simulink model "zynq_7000_tutorial_3"  (R2022a)
settings: Solver=FixedStepDiscrete  StartTime=0.0  StopTime=10.0  RelTol=1e-3
PostLoadFcn:
  | zynq7000.setModelProperties(bdroot)
undefined symbols (not defined in the file): AXI_VDMA, B, cam_init, G, init_cam, out1, out2, out3, OV5640, PS_GPIO, PS_IIC, R, read_cam_rgb, ScuGicInterruptController, VideoOutput
libraries: waijung2_utilities_lib x2, deeplib x1
Description:
  | This model is created using Waijung 2
  | (Version: 23.5a)
settings Model: Creator=Aimagin  LastModifiedBy=Chris
settings SolverCC: PositivePriorityOrder=on  AutoInsertRateTranBlk=on
settings OptimizationCC: DefaultParameterBehavior=Inlined  EnhancedBackFolding=on  PassReuseOutputArgsAs=Individual arguments  ZeroExternalMemoryAtStartup=off  ZeroInternalMemoryAtStartup=off  OptimizeBlockOrder=speed  DifferentSizesBufferReuse=on  OptimizationCustomize=off  EfficientTunableParamExpr=on
settings DebuggingCC: ParameterTunabilityLossMsg=error
settings HardwareCC: ProdBitPerPointer=32  ProdBitPerSizeT=32  ProdBitPerPtrDiffT=32  ProdLargestAtomicInteger=Long  ProdLargestAtomicFloat=Double  ProdWordSize=32  ProdHWDeviceType=ARM Compatible->ARM Cortex
settings SFSimCC: MATLABDynamicMemAlloc=off
settings RTWCC: Description=Waijung 2 ZYNQ7000 target  SystemTargetFile=zynq7000.tlc  TemplateMakefile=zynq7000.tmf  RetainRTWFile=on  TargetLang=C++  DLTargetLibrary=arm-compute  DLArmComputeArch=armv7
settings CodeAppCC: ForceParamTrailComments=on  IgnoreCustomStorageClasses=off  OperatorAnnotations=on  SimulinkDataObjDesc=on  SFDataObjDesc=on  InsertBlockDesc=on
settings STFCustomTargetCC: TargetLangStandard=C99 (ISO)  MultiwordLength=256  ModelReferenceCompliant=off  CombineOutputUpdateFcns=on  ERTCustomFileBanners=on  SupportContinuousTime=off  SupportNonInlinedSFcns=off  RemoveResetFunc=on  SupportVariableSizeSignals=on  MATLABClassNameForMDSCustomization=Simulink.SoftwareTarget.ERTCustomization  GRTInterface=off  SystemTargetFile=zynq7000.tlc
settings ERTTargetCC: TargetLangStandard=C99 (ISO)  ModelReferenceCompliant=off  ParMdlRefBuildCompliant=off  CompOptLevelCompliant=off  ConcurrentExecutionCompliant=off  SupportVariableSizeSignals=on  ModelStepFunctionPrototypeControlCompliant=off  CPPClassGenCompliant=off  UseToolchainInfoCompliant=off  InlinedParameterPlacement=NonHierarchical  ERTSrcFileBannerTemplate=zynq7000_code_template.cgt  ERTHdrFileBannerTemplate=zynq7000_code_template.cgt  ERTDataSrcFileTemplate=zynq7000_code_template.cgt  ERTDataHdrFileTemplate=zynq7000_code_template.cgt  ERTCustomFileTemplate=zynq7000_file_process.tlc

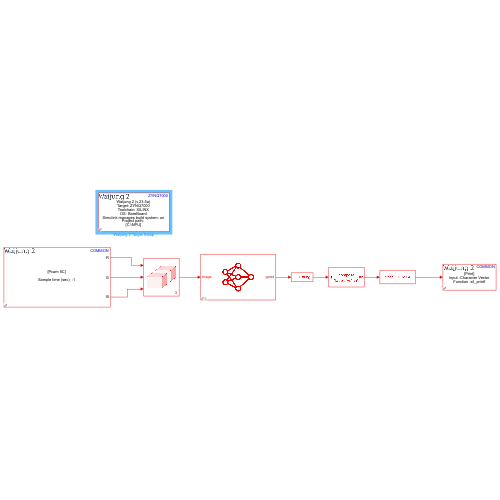
[thumbnail: Simulink's stored preview of the top-level diagram]
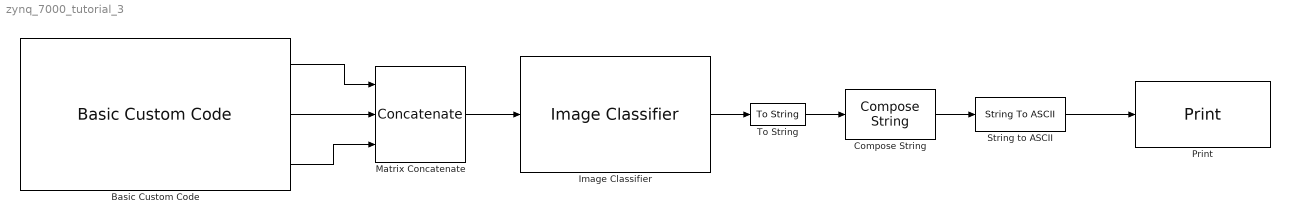
== system zynq_7000_tutorial_3 ==
  Basic Custom Code : waijung2_utilities_lib/Basic Custom Code  blockid=BasicCustomCode  maskdispname=Pcam 5C  inporttable={}  outporttable={ 'R', 'uint8', '1280x720'; 'G', 'uint8', '1280x720'; 'B', 'uint8', '1280x720' }  inputporttype=""  cinputportlabelstr="[\"\"]"  inputportcount=0  inputporttypeid=[-1]  outputporttype=uint8:1280x720,uint8:1280x720,uint8:1280x720  coutputportlabel=R,G,B  coutputportlabelstr="[\"R\",\"G\",\"B\"]"  outputportcount=3  outputporttypeid="[3  3  3]"  filepath="pwd,\"custom_lib\""  filenames=AXI_VDMA.c,AXI_VDMA.h,cam_init.c,cam_init.h,OV5640.c,OV5640.h,PS_GPIO.c,PS_GPIO.h,PS_IIC.c,PS_IIC.h,ScuGicInterruptController.h,VideoOutput.c,VideoOutput.h  incfilestrarray="[\"AXI_VDMA.h\",\"cam_init.h\",\"OV5640.h\",\"PS_GPIO.h\",\"PS_IIC.h\",\"ScuGicInterruptController.h\",\"VideoOutput.h\"]"  files=C:\NPU\custom_lib\AXI_VDMA.c,C:\NPU\custom_lib\AXI_VDMA.h,C:\NPU\custom_lib\cam_init.c,C:\NPU\custom_lib\cam_init.h,C:\NPU\custom_lib\OV5640.c,C:\NPU\custom_lib\OV5640.h,C:\NPU\custom_lib\PS_GPIO.c,C:\NPU\custom_lib\PS_GPIO.h,C:\NPU\custom_lib\PS_IIC.c,C:\NPU\custom_lib\PS_IIC.h,C:\NPU\custom_lib\ScuGicInterruptController.h,C:\NPU\custom_lib\VideoOutput.c,C:\NPU\custom_lib\VideoOutput.h  initialfuncallstr=init_cam();  outputfuncallstr=read_cam_rgb(out1, out2, out3);  inputportdiminfo=[]  outputportdiminfo="[1280     720  921600       3;1280     720  921600       3;1280     720  921600       3]"  enablecustomportlabel=on  sampletime=-1
      settings: SourceProductName=Waijung 2 Blockset
  Compose String : ComposeString  Format="\"label: %s\\r\\n\""
  Image Classifier : deeplib/Image Classifier  Network=Network from MATLAB function  NetworkFunction=mobilenetv2  NetworkFilePath=untitled.mat  MiniBatchSize=128  ResizeInput=on  Classification=on  Predictions=off  ForceInterpretedSim=off  PredictMode=All probabilities and labels  K=5
      settings: SourceProductBaseCode=NN
  Matrix Concatenate : Concatenate  NumInputs=3  Mode=Multidimensional array  ConcatenateDimension=3
  Print : waijung2_utilities_lib/Print  printfcn=xil_printf  strinput=Character Vector  sampletime=-1  blockid=Print  sampletimestr=2
      settings: SourceProductName=Waijung 2 Blockset
  String to ASCII : StringToASCII  OutputVectorSize=64
  To String : ToString
  wires:
  Basic Custom Code/1 -> Matrix Concatenate/1
  Basic Custom Code/2 -> Matrix Concatenate/2
  Basic Custom Code/3 -> Matrix Concatenate/3
  Matrix Concatenate/1 -> Image Classifier/1
  Image Classifier/1 -> To String/1
  To String/1 -> Compose String/1
  Compose String/1 -> String to ASCII/1
  String to ASCII/1 -> Print/1
